simulink model "Battery_Model_1cell_param_"  (R2021b)
settings: Solver=ode3  StartTime=0  StopTime=60000  FixedStep=10  RelTol=1e-3
undefined symbols (not defined in the file or in its folder): Cap, Cell_dev_mean, Cell_dev_sigma, Current_exp_high, n_cells, OCV1, OCV10, OCV2, OCV3, OCV4, OCV5, OCV6, OCV7, OCV8, OCV9, pCl1_High, pCl1_Low, pCl1_Mid, pCl2_High, pCl2_Low, pCl2_Mid, pCl3_High, pCl3_Low, pCl3_Mid, pCs1_High, pCs1_Low, pCs1_Mid, pCs2_High, pCs2_Low, pCs2_Mid, pCs3_High, pCs3_Low, pCs3_Mid, pRl1_High, pRl1_Low, pRl1_Mid, pRl2_High, pRl2_Low, pRl2_Mid, pRl3_High, pRl3_Low, pRl3_Mid, pRs1_High, pRs1_Low, pRs1_Mid, pRs2_High, pRs2_Low, pRs2_Mid, pRs3_High, pRs3_Low, pRs3_Mid, pRse1_High, pRse1_Low, pRse1_Mid, pRse2_High, pRse2_Low, pRse2_Mid, pRse3_High, pRse3_Low, pRse3_Mid ... (+6)
libraries: simulink x2, matrix_library x1
(part 2 of 2)

== matlab function Battery_Model_1cell_param_/Equivalent Circuit Model/Li_ion_Battery_Subsystem/Li_ion_Battery ==
  data: Val_in input; Val_out output; Param_in input; Rint input; dt input; CCorCV input; Test_Type input; I_in input; V_in input; P_in input; SOC_in input; I_balance input; V_out output; I_out output; SOC_out output; CCorCV_out output; W_resis output; Voc_cell output; Voc_pack output
function [Val_out, V_out, I_out ,SOC_out, CCorCV_out, W_resis, Voc_cell, Voc_pack]  = Li_ion_Battery(Val_in, Param_in, Rint,  dt,  CCorCV, Test_Type, I_in, V_in, P_in,  SOC_in, I_balance)
% function [Val_out, V_out, I_out ,SOC_out, V_min, V_max]  = Li_ion_max(Val_in, Param_in, R_int,  dt,  CCorCV, Test_Type, I_in, V_in, SOC_in, I_balance, OCV_pp)
%% Initialize Parameter Size
% Battery Parameters
n_max=32;
n_cell=Param_in(27);
E0=zeros(1,n_max);
R0=zeros(1,n_max);
R1=zeros(1,n_max);
R2=zeros(1,n_max);
C1=zeros(1,n_max);
C2=zeros(1,n_max);
SOC=zeros(1,n_max);
SOC_ini=zeros(1,n_max);  % If SOC is not given, we have to calculate the SOC value
SOC_out=zeros(1,n_max);  % If SOC is not given, we have to calculate the SOC value
CCorCV_out=0;
W_resis=zeros(1,n_max);
Voc_cell=zeros(1,n_max);
Voc_pack=0;

% Calculated Parameters
Vr=zeros(1,n_max);
Vrc1=zeros(1,n_max);
Vrc2=zeros(1,n_max);
V_out=zeros(1,n_max);
I_out=0;

% Recursive Parameters 
% These values are obtained from the previous step
Val_in=zeros(5,n_max)+Val_in;
Vrc1_ini=zeros(1,n_max)+Val_in(1,1:n_max);
Vrc2_ini=zeros(1,n_max)+Val_in(2,1:n_max);
SOC_diff=zeros(1,n_max)+Val_in(3,1:n_max);
I_in2=zeros(1,n_max)+Val_in(4,1:n_max);
V_pack=zeros(1)+Val_in(5,1); 
Val_out=zeros(5,n_max);


% Reset button on!
% if (CCorCV==4)
%     Vrc1_ini=zeros(1,n_max);
%     Vrc2_ini=zeros(1,n_max);
%     SOC_diff=zeros(1,n_max);
%     I_in2=zeros(1,n_max);
%     V_pack=zeros(1);
%     CCorCV=1;     % Convert to CC rest mode
%     Test_Type=0;
% end

if (Test_Type==4)
    Vrc1_ini=zeros(1,n_max);
    Vrc2_ini=zeros(1,n_max);
    SOC_diff=zeros(1,n_max);
    I_in2=zeros(1,n_max);
    V_pack=zeros(1);
    CCorCV=1;     % Convert to CC rest mode
    Test_Type=0;
end



%% Set Battery Parameters
% Battery Parameters
Cap=Param_in(26);
Ctot=3600*Cap;

OCV1=	Param_in(1);
OCV2=	Param_in(2);
OCV3=	Param_in(3);
OCV4=	Param_in(4);
OCV5=	Param_in(5);
OCV6=	Param_in(6);
OCV7=	Param_in(7);
OCV8=	Param_in(8);
OCV9=	Param_in(9);
OCV10=	Param_in(10);
pRse1=	Param_in(11);
pRse2=	Param_in(12);
pRse3=	Param_in(13);
pRs1=	Param_in(14);
pRs2=	Param_in(15);
pRs3=	Param_in(16);
pRl1=	Param_in(17);
pRl2=	Param_in(18);
pRl3=	Param_in(19);
pCs1=	Param_in(20);
pCs2=	Param_in(21);
pCs3=	Param_in(22);
pCl1=	Param_in(23);
pCl2=	Param_in(24);
pCl3=	Param_in(25);



%% Calculate Battery Parameters
% CCorCV=0 then CC/CV(This varies wrt. the lower and upper bound voltage limits)
% CCorCV=1 then CC(constant current)
% CCorCV=2 then CV(constant voltage)
% Test_Type 0:Rest, 1:Charge, 2:Discharge

% Find out whether CC or CV should be applied.
if (CCorCV==0)
    if (Test_Type==0)  % Rest?
        CCorCV=1;      % CC Mode with 0    
    elseif (V_pack>=V_in-(10e-10) && Test_Type==1 && V_pack~=0) % Charge CV? with the error boundary
        CCorCV=2;
    elseif (V_pack<=V_in+(10e-10) && Test_Type==2 && V_pack~=0) % Discharge CV? with the error boundary
        CCorCV=2;      
    else
        CCorCV=1; % CC
    end
end


















%% Caculate the Voltage and SOC values of the battery pack
%%%%%%%%% CC mode Calculation
if (CCorCV==1)
    
%%%%%%%%% Rest Charge or Discharge mode
    if (Test_Type==0) % Rest?
        I_in=0; 
    elseif (Test_Type==1) % Charge?
        I_in=abs(I_in);
    else 
        I_in=-abs(I_in); % Discharge?
    end
    
for j=1:n_cell
%%%%%%%%% If only SOC ini is given
SOC_ini(j)=SOC_in; 
%%%%%%%%% Overcharged or discharged
if ((SOC_ini(j)+SOC_diff(j)>1.05 && I_in>0) || (SOC_ini(j)+SOC_diff(j)< 0.01 && I_in<0))
    I_in=0;
end
if ((SOC_ini(j)+SOC_diff(j)>1.05 && I_balance(j)>0) || (SOC_ini(j)+SOC_diff(j)< 0.01 && I_balance(j)<0))
    I_balance(j)=0;
end
SOC_diff(j)=SOC_diff(j)+dt*(I_in+I_balance(j))/Ctot;
SOC(j)=SOC_ini(j)+SOC_diff(j);
Val_out(3,j)=SOC_diff(j);

%%%%%%%%% If SOC  is given
% SOC(j)=SOC_in;   

E0(j) = OCV1 * exp(OCV2 * SOC(j)) + OCV3 * SOC(j) ^ 7 + OCV4 * SOC(j) ^ 6 + OCV5 * SOC(j) ^ 5 + OCV6 * SOC(j) ^ 4 + OCV7 * SOC(j) ^ 3 + OCV8 * SOC(j) ^ 2 + OCV9 * SOC(j) + OCV10;
% E0(j) = interp1(OCV_pp(2,:),OCV_pp(1,:),SOC(j),'spline'); % Use look up table value
R0(j) = pRse1*exp(pRse2*SOC(j))+pRse3+Rint(j);
R1(j) = pRs1*exp(pRs2*SOC(j))+pRs3;
C1(j) = pCs1*exp(pCs2*SOC(j))+pCs3;
R2(j) = pRl1*exp(pRl2*SOC(j))+pRl3;
C2(j) = pCl1*exp(pCl2*SOC(j))+pCl3;

Vr(j)   = (I_in+I_balance(j)) * R0(j);
Vrc1(j) = Vrc1_ini(j) * exp(-dt/(R1(j)*C1(j))) + (I_in+I_balance(j)) * R1(j) * (1-exp(-dt/(R1(j)*C1(j)))); 
Vrc2(j) = Vrc2_ini(j) * exp(-dt/(R2(j)*C2(j))) + (I_in+I_balance(j)) * R2(j) * (1-exp(-dt/(R2(j)*C2(j)))); 
V_out(j) = E0(j)+Vr(j)+Vrc1(j)+Vrc2(j);
Val_out(1,j)=Vrc1(j);
Val_out(2,j)=Vrc2(j);
Val_out(4,j)=I_in+I_balance(j);
I_out=I_in;

W_resis(j)=abs((I_out+I_balance(j))*(V_out(j)-E0(j)));
end    


















%%%%%%%%%%%%%%%%%%%%%%%%%%%%%%%%%%%%%%%%%
%%%%%%%%% CV mode Calculation
elseif(CCorCV==2)   
phi_temp=0;
gamma_temp=0;

for j=1:n_cell   
%%%%%%%%% If only SOC ini is given
SOC_ini(j)=SOC_in; 
SOC_diff(j)=SOC_diff(j)+dt*(Val_in(4,j))/Ctot;
SOC(j)=SOC_ini(j)+SOC_diff(j);
Val_out(3,j)=SOC_diff(j);

%%%%%%%%% If SOC  is given
% SOC(j)=SOC_in;   

E0(j) = OCV1 * exp(OCV2 * SOC(j)) + OCV3 * SOC(j) ^ 7 + OCV4 * SOC(j) ^ 6 + OCV5 * SOC(j) ^ 5 + OCV6 * SOC(j) ^ 4 + OCV7 * SOC(j) ^ 3 + OCV8 * SOC(j) ^ 2 + OCV9 * SOC(j) + OCV10;
% E0(j) = interp1(OCV_pp(2,:),OCV_pp(1,:),SOC(j),'spline'); % Use look up table value
R0(j) = pRse1*exp(pRse2*SOC(j))+pRse3+Rint(j);
R1(j) = pRs1*exp(pRs2*SOC(j))+pRs3;
C1(j) = pCs1*exp(pCs2*SOC(j))+pCs3;
R2(j) = pRl1*exp(pRl2*SOC(j))+pRl3;
C2(j) = pCl1*exp(pCl2*SOC(j))+pCl3;  

phi_temp=(R0(j)+R1(j)*(1-exp(-dt/(R1(j)*C1(j))))+R2(j)*(1-exp(-dt/(R2(j)*C2(j)))))+phi_temp;
gamma_temp=E0(j)+Vrc1_ini(j)*(exp(-dt/(R1(j)*C1(j))))+Vrc2_ini(j)*(exp(-dt/(R2(j)*C2(j))))+(R0(j)+R1(j)*(1-exp(-dt/(R1(j)*C1(j))))+R2(j)*(1-exp(-dt/(R2(j)*C2(j)))))*I_balance(j)+gamma_temp;
end  

%%%%%%%%% Calculate I_in
%%%%%%%%% Rest Charge or Discharge mode
    if (Test_Type==0) % Rest?
        I_in=0; 
    else
        I_in=(V_in-gamma_temp)/phi_temp;
    end

%%%%%%%%% Overcharged or discharged
if ((SOC_ini(j)+SOC_diff(j)>1.05 && I_in>0) || (SOC_ini(j)+SOC_diff(j)< 0.01 && I_in<0))
    I_in=0;
end
if ((SOC_ini(j)+SOC_diff(j)>1.05 && I_balance(j)>0) || (SOC_ini(j)+SOC_diff(j)< 0.01 && I_balance(j)<0))
    I_balance(j)=0;
end

for j=1:n_cell 
Vr(j)   = (I_in+I_balance(j)) * R0(j);
Vrc1(j) = Vrc1_ini(j) * exp(-dt/(R1(j)*C1(j))) + (I_in+I_balance(j)) * R1(j) * (1-exp(-dt/(R1(j)*C1(j)))); 
Vrc2(j) = Vrc2_ini(j) * exp(-dt/(R2(j)*C2(j))) + (I_in+I_balance(j)) * R2(j) * (1-exp(-dt/(R2(j)*C2(j)))); 
V_out(j) = E0(j)+Vr(j)+Vrc1(j)+Vrc2(j);
Val_out(1,j)=Vrc1(j);
Val_out(2,j)=Vrc2(j);
Val_out(4,j)=I_in+I_balance(j);
I_out=I_in;

W_resis(j)=abs((I_out+I_balance(j))*(V_out(j)-E0(j)));
end











%%%%%%%%% CP mode Calculation
elseif (CCorCV==3)
phi_temp=0;
gamma_temp=0;

for j=1:n_cell   
%%%%%%%%% If only SOC ini is given
SOC_ini(j)=SOC_in; 
SOC_diff(j)=SOC_diff(j)+dt*(Val_in(4,j))/Ctot;
SOC(j)=SOC_ini(j)+SOC_diff(j);
Val_out(3,j)=SOC_diff(j);

%%%%%%%%% If SOC  is given
% SOC(j)=SOC_in;   

E0(j) = OCV1 * exp(OCV2 * SOC(j)) + OCV3 * SOC(j) ^ 7 + OCV4 * SOC(j) ^ 6 + OCV5 * SOC(j) ^ 5 + OCV6 * SOC(j) ^ 4 + OCV7 * SOC(j) ^ 3 + OCV8 * SOC(j) ^ 2 + OCV9 * SOC(j) + OCV10;
% E0(j) = interp1(OCV_pp(2,:),OCV_pp(1,:),SOC(j),'spline'); % Use look up table value
R0(j) = pRse1*exp(pRse2*SOC(j))+pRse3+Rint(j);
R1(j) = pRs1*exp(pRs2*SOC(j))+pRs3;
C1(j) = pCs1*exp(pCs2*SOC(j))+pCs3;
R2(j) = pRl1*exp(pRl2*SOC(j))+pRl3;
C2(j) = pCl1*exp(pCl2*SOC(j))+pCl3;  

phi_temp=(R0(j)+R1(j)*(1-exp(-dt/(R1(j)*C1(j))))+R2(j)*(1-exp(-dt/(R2(j)*C2(j)))))+phi_temp;
gamma_temp=E0(j)+Vrc1_ini(j)*(exp(-dt/(R1(j)*C1(j))))+Vrc2_ini(j)*(exp(-dt/(R2(j)*C2(j))))+(R0(j)+R1(j)*(1-exp(-dt/(R1(j)*C1(j))))+R2(j)*(1-exp(-dt/(R2(j)*C2(j)))))*I_balance(j)+gamma_temp;
end  
    

%%%%%%%%% Calculate I_in
%%%%%%%%% Rest Charge or Discharge mode
    if (Test_Type==0) % Rest?
        I_in=0; 
    elseif (Test_Type==1) % Charge?
        I_in=(-gamma_temp+sqrt(gamma_temp^2-4*phi_temp*(-abs(P_in))))/(2*phi_temp);
    else 
        I_in=(-gamma_temp+sqrt(gamma_temp^2-4*phi_temp*(abs(P_in))))/(2*phi_temp); % Discharge?
    end


%%%%%%%%% Overcharged or discharged
if ((SOC_ini(j)+SOC_diff(j)>1.05 && I_in>0) || (SOC_ini(j)+SOC_diff(j)< 0.01 && I_in<0))
    I_in=0;
end
if ((SOC_ini(j)+SOC_diff(j)>1.05 && I_balance(j)>0) || (SOC_ini(j)+SOC_diff(j)< 0.01 && I_balance(j)<0))
    I_balance(j)=0;
end

for j=1:n_cell 
Vr(j)   = (I_in+I_balance(j)) * R0(j);
Vrc1(j) = Vrc1_ini(j) * exp(-dt/(R1(j)*C1(j))) + (I_in+I_balance(j)) * R1(j) * (1-exp(-dt/(R1(j)*C1(j)))); 
Vrc2(j) = Vrc2_ini(j) * exp(-dt/(R2(j)*C2(j))) + (I_in+I_balance(j)) * R2(j) * (1-exp(-dt/(R2(j)*C2(j)))); 
V_out(j) = E0(j)+Vr(j)+Vrc1(j)+Vrc2(j);
Val_out(1,j)=Vrc1(j);
Val_out(2,j)=Vrc2(j);
Val_out(4,j)=I_in+I_balance(j);
I_out=I_in;

W_resis(j)=abs((I_out+I_balance(j))*(V_out(j)-E0(j)));
end
















end















for j=1:n_cell 
SOC_out(j)=SOC(j); 
end

%%%%%%%%% Battery Output Values
% V_min=min(V_out(1:n_cell));
% V_max=max(V_out(1:n_cell));
Voc_pack=sum(E0(1:n_cell));
Voc_cell=E0;
V_pack=sum(V_out(1:n_cell));

Val_out(5,1)=V_pack;
CCorCV_out=CCorCV;

end

== matlab function Battery_Model_1cell_param_/Equivalent Circuit Model/Li_ion_Battery_Subsystem/Param_in/2D interpolation ==
  data: T_pack input; Temp1 input; Param_out output; Temp2 input; Temp3 input; Param1 input; Param2 input; Param3 input
function Param_out= fcn(T_pack, Temp1, Temp2, Temp3, Param1, Param2, Param3)
%#codegen
% if (T_pack<T_amb)
%     T_pack=T_amb;
% end

if Temp1==Temp2
    Temp2=Temp2+10e-5;
end
if Temp2==Temp3
    Temp3=Temp3+10e-5;
end
if Temp1==Temp3
    Temp3=Temp3+10e-5;
end



x= [Temp1, Temp2, Temp3];
v= [Param1'; Param2'; Param3'];
vq = interp1(x,v,T_pack,'linear','extrap');

% Extrapolation 값이 이상하여 아래와 같이 extrapolation 대신 clip을 해주는 함수 삽입
if T_pack<Temp1
    vq=Param1';
elseif T_pack>Temp3
    vq=Param3';
end


Param_out=vq';

== matlab function Battery_Model_1cell_param_/Equivalent Circuit Model/Li_ion_Battery_Subsystem/Param_in/Internal Resistance Calc ==
  data: Param_in input; Rint output
function Rint  = Initialise_function(Param_in)
%#codegen
% This method approximates the normal distribution curve
n_max=32;
n_cell=Param_in(1);

Rint=zeros(1,n_max);
a_dist=zeros(1,n_max);

% For the z transformed probability Density function
% theta = (1/sqrt(2*pi))*exp(-z^2/2)) where z=(x-mean)/alpha
pRin1= Param_in(2);  % Mean
pRin2= Param_in(3);  % Variance

Z=-3:0.2:3;
f_cd=zeros(1,length(Z));
f_nd=(1/sqrt(2*pi))*exp(-(Z).^2/(2));
f_cd(1)=(1-0.997300203914589)/2;
for i=2:length(f_nd)
    f_cd(i)=f_cd(i-1)+(f_nd(i)+f_nd(i-1))/2*(Z(i)-Z(i-1));
end

% with in 90% range (0.05<val<0.95)
for i=1:n_cell
a_dist(i)=0.05+0.9/(n_cell-1)*(i-1);
end

% Linear interpolation and R_in calculation
for j=1:length(a_dist)
    for i=1:length(f_cd)-1
        if (f_cd(i+1)>=a_dist(j) && a_dist(j)>f_cd(i))
            Rint(j)=((a_dist(j)-f_cd(i))*(Z(i+1)-Z(i))/(f_cd(i+1)-f_cd(i))+Z(i))*pRin2+pRin1;% Multiplied by the Standard deviation and added the mean value
        end
    end
end

== matlab function Battery_Model_1cell_param_/Equivalent Circuit Model/Li_ion_Battery_Subsystem/Param_in/Temp Calc ==
  data: T_Ini input; T_amb input; T_out output; m input; A input; h input; Cp input; E input; SB_const input; dVdT input; W_resis input; I_pack input; T_pack input; dt input; W_entropy output; W_convection output; W_radiation output; W_tot output; n_cell input; Test_Type input; Step_Count input
function [T_out,W_entropy, W_convection, W_radiation, W_tot] = temp_model(T_Ini, T_amb, m, A, h, Cp, E, SB_const, dVdT, W_resis, I_pack, T_pack, dt,n_cell, Test_Type, Step_Count)
%#codegen
T_amb=T_amb+273;
T_pack=T_pack+273;

if (Step_Count<2)
    T_pack=T_Ini+273;
end


W_entropy=I_pack*T_pack*dVdT;
W_convection=h*A*(T_pack-T_amb);
W_radiation=E*SB_const*A*(T_pack^4-T_amb^4);

W_tot=W_resis+W_entropy-W_convection-W_radiation;

delta_T=(W_tot/(m*Cp)*dt)/(n_cell);

T_out=T_pack+delta_T-273;


% Reset on
% if (Test_Mode ==4)
%     T_out=T_amb-273;
% end

if (Test_Type ==4)
    T_out=T_Ini-273;
end
